simulink model "MaxPilot"  (R2026a)
settings: Solver=VariableStepAuto  StopTime=inf
undefined symbols (not defined in the file or in its folder): f
libraries: instrumentlib x8, slpidlib x4, SignalEditorBlockLib x1
settings Model: Creator=max  LastModifiedBy=Owner

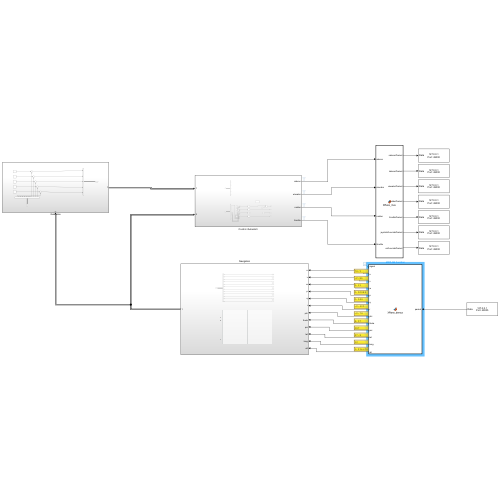
[thumbnail: Simulink's stored preview of the top-level diagram]
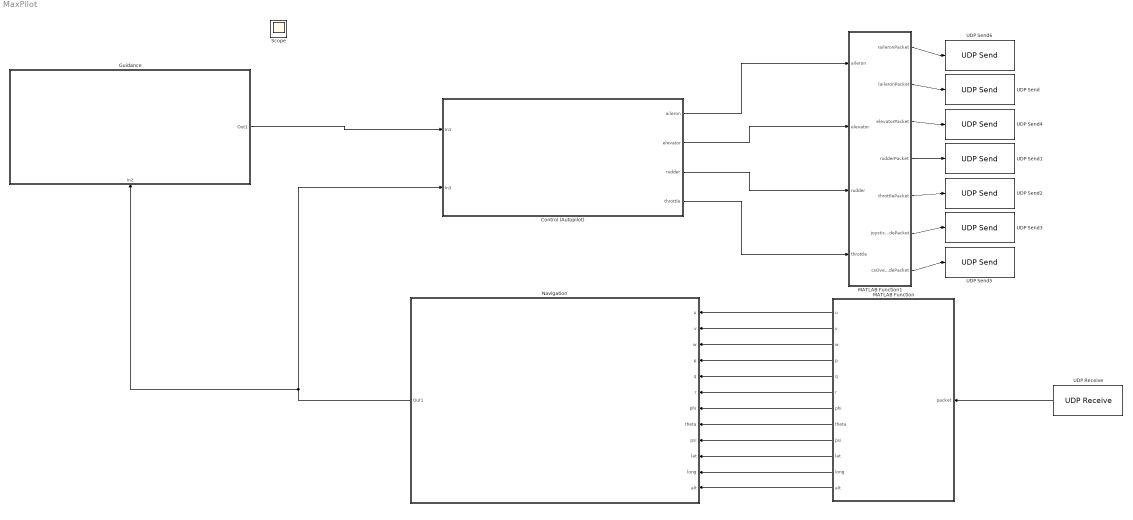
== system MaxPilot ==
  Control (Autopilot) : Subsystem
  Guidance : Subsystem
      settings: PortSchema="{\"entries\":[{\"content\":{\"sides\":[{\"content\":{},\"type\":\"ConnectorPlacement.EquallySpacedRectSide\",\"uuid\":\"e11f845c-727a-4623-8abb-a86b842d9894\"},{\"content\":{\"connectorIds\":[\"Out1\"],\"side\":\"RIGHT\"},\"type\":\"ConnectorPlacement.EquallySpacedRectSide\",\"uuid\":\"0ead8184-70d2-4c1b-98dc-64e560e2a903\"},{\"content\":{\"side\":\"TOP\"},\"type\":\"ConnectorPlacement.EquallySpacedRectSide\",\"uuid\":\"faab937e-1283-4214-83c9-3a230b74f371\"},{\"content\":{\"connectorIds\":[\"In1\"],\"side\":\"BOTTOM\"},\"type\":\"ConnectorPlacement.EquallySpacedRectSide\",\"uuid\":\"89b0e162-5b11-45eb-99f5-a61c863778c0\"}]},\"type\":\"ConnectorPlacement.EquallySpacedConnector\",\"uuid\":\"efd43e26-ed77-40df-bb71-45bc413bd349\"}],\"packageUris\":[\"http://schema.mathworks.com/mf0/Connector/R2020b\"],\"version\":\"1.0\"}"
  MATLAB Function : MATLAB Function  TreatAsAtomicUnit=on
  MATLAB Function1 : MATLAB Function  TreatAsAtomicUnit=on
  Navigation : Subsystem
  UDP Receive : instrumentlib/UDP Receive  LocalAddress=127.0.0.1  LocalPort=49005  EnablePortSharing=off  Host=localhost  Port=9090  GetLatestData=on  DataSize=[ 185, 1 ]  DataType=uint8  ASCIIFormatting=%f,  Terminator=LF  CustomTerminator=10  ByteOrder=big-endian  EnableBlockingMode=on  Timeout=10  SampleTime=0.02  SimulateUsing=Interpreted execution
  UDP Send{,1..6} (7 alike) : instrumentlib/UDP Send  Host=127.0.0.1  Port=49000  LocalAddress=0.0.0.0  LocalPort=-1  EnablePortSharing=off  OutputDatagramPacketSize=509  ByteOrder=big-endian  EnableBlockingMode=on  SimulateUsing=Interpreted execution
  Scope : Scope
      settings: ActiveDisplayYMinimum=-1  ActiveDisplayYMaximum=1
  wires:
  Guidance/1(Out1) -> Control (Autopilot)/1(In1)
  Navigation/1(Out1) -> Control (Autopilot)/2(In3), Guidance/1(In2)
  UDP Receive/1 -> MATLAB Function/1(packet)
  MATLAB Function1/2(laileronPacket) -> UDP Send/1
  MATLAB Function1/3(elevatorPacket) -> UDP Send4/1
  MATLAB Function1/5(throttlePacket) -> UDP Send2/1
  MATLAB Function1/6(joystickOverridePacket) -> UDP Send3/1
  MATLAB Function1/4(rudderPacket) -> UDP Send1/1
  MATLAB Function1/7(csOverridePacket) -> UDP Send5/1
  MATLAB Function1/1(raileronPacket) -> UDP Send6/1
  Control (Autopilot)/1(aileron) -> MATLAB Function1/1(aileron)
  Control (Autopilot)/2(elevator) -> MATLAB Function1/2(elevator)
  Control (Autopilot)/3(rudder) -> MATLAB Function1/3(rudder)
  Control (Autopilot)/4(throttle) -> MATLAB Function1/4(throttle)
  MATLAB Function/2(v) -> Navigation/2(v)
  MATLAB Function/3(w) -> Navigation/3(w)
  MATLAB Function/4(p) -> Navigation/4(p)
  MATLAB Function/5(q) -> Navigation/5(q)
  MATLAB Function/6(r) -> Navigation/6(r)
  MATLAB Function/7(phi) -> Navigation/7(phi)
  MATLAB Function/8(theta) -> Navigation/8(theta)
  MATLAB Function/9(psi) -> Navigation/9(psi)
  MATLAB Function/10(lat) -> Navigation/10(lat)
  MATLAB Function/11(long) -> Navigation/11(long)
  MATLAB Function/12(alt) -> Navigation/12(alt)
  MATLAB Function/1(u) -> Navigation/1(u)

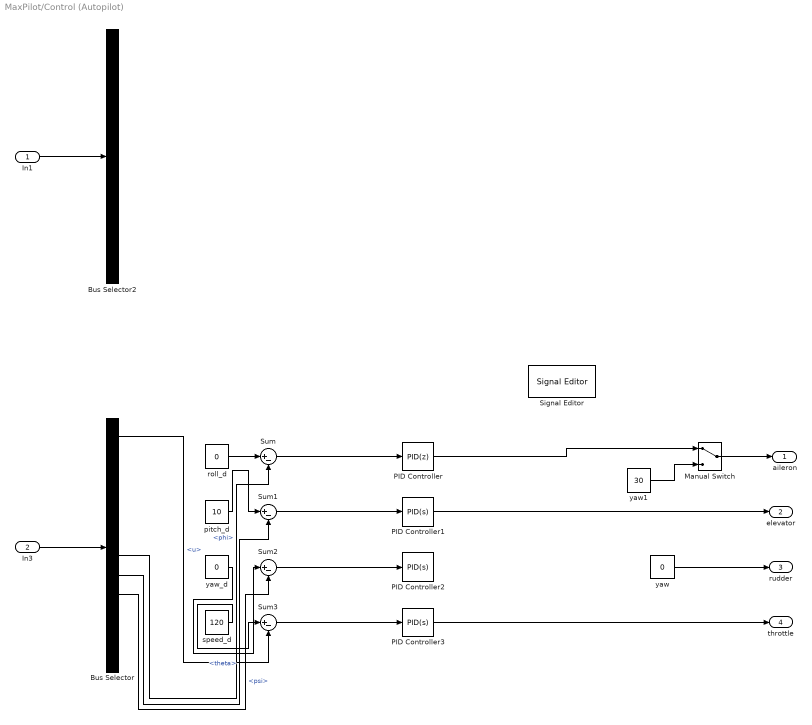
== system MaxPilot/Control (Autopilot) ==
  In1 : Inport
  In3 : Inport  Port=2
  Bus Selector : BusSelector  OutputSignals=u,v,w,p,q,r,phi,theta,psi,lat,long,alt
  Bus Selector2 : BusSelector  OutputSignals=psi_e,North_e,East_e,alt_e,u_e
  Manual Switch : ManualSwitch
  PID Controller : slpidlib/PID Controller  Controller=PID  Form=Parallel  TimeDomain=Discrete-time  UseExternalTs=off  SampleTime=-1  IntegratorMethod=Forward Euler  FilterMethod=Forward Euler  ControllerParametersSource=internal  P=1  I=0  UseKiTs=off  D=0  UseExternalDerivativeSource=off  N=100  UseFilter=on  TunerSelectOption=Frequency Response Based  ZeroCross=off  InitialConditionSource=internal  InitialConditionForIntegrator=0  InitialConditionForFilter=0  DifferentiatorICPrevScaledInput=0  ExternalReset=none  TrackingMode=off  Kt=1  LimitOutput=on  SatLimitsSource=internal  UpperSaturationLimit=10  LowerSaturationLimit=-10  LinearizeAsGain=on  AntiWindupMode=none  Kb=1  LimitIntegrator=off  UpperIntegratorSaturationLimit=inf  LowerIntegratorSaturationLimit=-inf  POutMin=[]  POutMax=[]  IOutMin=[]  IOutMax=[]  DOutMin=[]  DOutMax=[]  NOutMin=[]  NOutMax=[]  SumOutMin=[]  SumOutMax=[]  SaturationOutMin=[]  SaturationOutMax=[]  PParamMin=[]  PParamMax=[]  IParamMin=[]  IParamMax=[]  DParamMin=[]  DParamMax=[]  NParamMin=[]  NParamMax=[]  KbParamMin=[]  KbParamMax=[]  KtParamMin=[]  KtParamMax=[]  KbOutMin=[]  KbOutMax=[]  KtOutMin=[]  KtOutMax=[]  IntegratorOutMin=[]  IntegratorOutMax=[]  FilterOutMin=[]  FilterOutMax=[]  SumI1OutMin=[]  SumI1OutMax=[]  SumI2OutMin=[]  SumI2OutMax=[]  SumI3OutMin=[]  SumI3OutMax=[]  SumI4OutMin=[]  SumI4OutMax=[]  SumDOutMin=[]  SumDOutMax=[]  DifferentiatorOutMin=[]  DifferentiatorOutMax=[]  FilterDiffOutCoefMin=[]  FilterDiffOutCoefMax=[]  ReciprocalOutMin=[]  ReciprocalOutMax=[]  SumDenOutMin=[]  SumDenOutMax=[]  SumNumOutMin=[]  SumNumOutMax=[]  DivideOutMin=[]  DivideOutMax=[]  UdiffTsProdOutMin=[]  UdiffTsProdOutMax=[]  NTsProdOutMin=[]  NTsProdOutMax=[]  UintegralTsProdOutMin=[]  UintegralTsProdOutMax=[]  UngainTsProdOutMin=[]  UngainTsProdOutMax=[]  ClampingZeroOutDataTypeStr=Inherit: Inherit via back propagation  ClampingZeroOutMin=[]  ClampingZeroOutMax=[]  FilterDenConstantOutDataTypeStr=Inherit: Inherit via back propagation  FilterDenConstantOutMin=[]  FilterDenConstantOutMax=[]  PCopyOutDataTypeStr=Inherit: Inherit via back propagation  PCopyOutMin=[]  PCopyOutMax=[]  NCopyOutDataTypeStr=Inherit: Inherit via back propagation  NCopyOutMin=[]  NCopyOutMax=[]  IntegratorContinuousStateAttributes=''  IntegratorStateMustResolveToSignalObject=off  IntegratorRTWStateStorageClass=Auto  FilterContinuousStateAttributes=''  FilterStateMustResolveToSignalObject=off  FilterRTWStateStorageClass=Auto  ParallelPVariant=InternalParameters  IdealPVariant=Disabled  IVariant=InternalParameters  DVariant=InternalParameters  IntegratorVariant=Discrete  SatVariant=Enabled  AWVariant=Passthrough  PCopyVariant=Disabled  TRVariant=Disabled  FdbkBlocksVariant=Forward  IdealPFdbkVariant=Disabled  SatFdbkVariant=Disabled  DerivativeFilterVariant=ForwardEulerFilter  NVariant=InternalParameters  NCopyVariant=Disabled  FilterICVariant=InternalICsFilter  IntegratorICVariant=InternalICs  ExternalResetVariant=Disabled  TRSumVariant=Passthrough  SumFdbkVariant=Disabled  SumVariant=Sum_PID  TsampFilterVariant=InternalTs  TsampNgainVariant=Passthrough  TsampIntegralVariant=Disabled_SignalSpec  ExternalSaturationOutDataTypeStr=Inherit: Same as second input  DerivativeSourceVariant=ErrorSignal  PreIntVariant=InternalPreInt
  PID Controller1 : slpidlib/PID Controller  Controller=PID  Form=Parallel  TimeDomain=Continuous-time  UseExternalTs=off  SampleTime=-1  IntegratorMethod=Forward Euler  FilterMethod=Forward Euler  ControllerParametersSource=internal  P=0.75  I=0  UseKiTs=off  D=0  UseExternalDerivativeSource=off  N=100  UseFilter=on  TunerSelectOption=Transfer Function Based (PID Tuner App)  InitialConditionSource=internal  InitialConditionForIntegrator=0  InitialConditionForFilter=0  DifferentiatorICPrevScaledInput=0  ExternalReset=none  TrackingMode=off  Kt=1  LimitOutput=on  SatLimitsSource=internal  UpperSaturationLimit=20  LowerSaturationLimit=-25  LinearizeAsGain=on  AntiWindupMode=none  Kb=1  LimitIntegrator=off  UpperIntegratorSaturationLimit=inf  LowerIntegratorSaturationLimit=-inf  POutMin=[]  POutMax=[]  IOutMin=[]  IOutMax=[]  DOutMin=[]  DOutMax=[]  NOutMin=[]  NOutMax=[]  SumOutMin=[]  SumOutMax=[]  SaturationOutMin=[]  SaturationOutMax=[]  PParamMin=[]  PParamMax=[]  IParamMin=[]  IParamMax=[]  DParamMin=[]  DParamMax=[]  NParamMin=[]  NParamMax=[]  KbParamMin=[]  KbParamMax=[]  KtParamMin=[]  KtParamMax=[]  KbOutMin=[]  KbOutMax=[]  KtOutMin=[]  KtOutMax=[]  IntegratorOutMin=[]  IntegratorOutMax=[]  FilterOutMin=[]  FilterOutMax=[]  SumI1OutMin=[]  SumI1OutMax=[]  SumI2OutMin=[]  SumI2OutMax=[]  SumI3OutMin=[]  SumI3OutMax=[]  SumI4OutMin=[]  SumI4OutMax=[]  SumDOutMin=[]  SumDOutMax=[]  DifferentiatorOutMin=[]  DifferentiatorOutMax=[]  FilterDiffOutCoefMin=[]  FilterDiffOutCoefMax=[]  ReciprocalOutMin=[]  ReciprocalOutMax=[]  SumDenOutMin=[]  SumDenOutMax=[]  SumNumOutMin=[]  SumNumOutMax=[]  DivideOutMin=[]  DivideOutMax=[]  UdiffTsProdOutMin=[]  UdiffTsProdOutMax=[]  NTsProdOutMin=[]  NTsProdOutMax=[]  UintegralTsProdOutMin=[]  UintegralTsProdOutMax=[]  UngainTsProdOutMin=[]  UngainTsProdOutMax=[]  ClampingZeroOutDataTypeStr=Inherit: Inherit via back propagation  ClampingZeroOutMin=[]  ClampingZeroOutMax=[]  FilterDenConstantOutDataTypeStr=Inherit: Inherit via back propagation  FilterDenConstantOutMin=[]  FilterDenConstantOutMax=[]  PCopyOutDataTypeStr=Inherit: Inherit via back propagation  PCopyOutMin=[]  PCopyOutMax=[]  NCopyOutDataTypeStr=Inherit: Inherit via back propagation  NCopyOutMin=[]  NCopyOutMax=[]  IntegratorContinuousStateAttributes=''  IntegratorStateMustResolveToSignalObject=off  IntegratorRTWStateStorageClass=Auto  FilterContinuousStateAttributes=''  FilterStateMustResolveToSignalObject=off  FilterRTWStateStorageClass=Auto  ParallelPVariant=InternalParameters  IdealPVariant=Disabled  IVariant=InternalParameters  DVariant=InternalParameters  IntegratorVariant=Continuous  SatVariant=Enabled  AWVariant=Passthrough  PCopyVariant=Disabled  TRVariant=Disabled  FdbkBlocksVariant=Forward  IdealPFdbkVariant=Disabled  SatFdbkVariant=Disabled  DerivativeFilterVariant=ContFilter  NVariant=InternalParameters  NCopyVariant=Disabled  FilterICVariant=InternalICsFilter  IntegratorICVariant=InternalICs  ExternalResetVariant=Disabled  TRSumVariant=Passthrough  SumFdbkVariant=Disabled  SumVariant=Sum_PID  TsampFilterVariant=InternalTs  TsampNgainVariant=Passthrough  TsampIntegralVariant=Disabled_SignalSpec  ExternalSaturationOutDataTypeStr=Inherit: Same as second input  DerivativeSourceVariant=ErrorSignal  PreIntVariant=InternalPreInt
  PID Controller2 : slpidlib/PID Controller  Controller=PID  Form=Parallel  TimeDomain=Continuous-time  UseExternalTs=off  SampleTime=-1  IntegratorMethod=Forward Euler  FilterMethod=Forward Euler  ControllerParametersSource=internal  P=1  I=0  UseKiTs=off  D=0  UseExternalDerivativeSource=off  N=100  UseFilter=on  TunerSelectOption=Transfer Function Based (PID Tuner App)  InitialConditionSource=internal  InitialConditionForIntegrator=0  InitialConditionForFilter=0  DifferentiatorICPrevScaledInput=0  ExternalReset=none  TrackingMode=off  Kt=1  LimitOutput=on  SatLimitsSource=internal  UpperSaturationLimit=15  LowerSaturationLimit=-15  LinearizeAsGain=on  AntiWindupMode=none  Kb=1  LimitIntegrator=off  UpperIntegratorSaturationLimit=inf  LowerIntegratorSaturationLimit=-inf  POutMin=[]  POutMax=[]  IOutMin=[]  IOutMax=[]  DOutMin=[]  DOutMax=[]  NOutMin=[]  NOutMax=[]  SumOutMin=[]  SumOutMax=[]  SaturationOutMin=[]  SaturationOutMax=[]  PParamMin=[]  PParamMax=[]  IParamMin=[]  IParamMax=[]  DParamMin=[]  DParamMax=[]  NParamMin=[]  NParamMax=[]  KbParamMin=[]  KbParamMax=[]  KtParamMin=[]  KtParamMax=[]  KbOutMin=[]  KbOutMax=[]  KtOutMin=[]  KtOutMax=[]  IntegratorOutMin=[]  IntegratorOutMax=[]  FilterOutMin=[]  FilterOutMax=[]  SumI1OutMin=[]  SumI1OutMax=[]  SumI2OutMin=[]  SumI2OutMax=[]  SumI3OutMin=[]  SumI3OutMax=[]  SumI4OutMin=[]  SumI4OutMax=[]  SumDOutMin=[]  SumDOutMax=[]  DifferentiatorOutMin=[]  DifferentiatorOutMax=[]  FilterDiffOutCoefMin=[]  FilterDiffOutCoefMax=[]  ReciprocalOutMin=[]  ReciprocalOutMax=[]  SumDenOutMin=[]  SumDenOutMax=[]  SumNumOutMin=[]  SumNumOutMax=[]  DivideOutMin=[]  DivideOutMax=[]  UdiffTsProdOutMin=[]  UdiffTsProdOutMax=[]  NTsProdOutMin=[]  NTsProdOutMax=[]  UintegralTsProdOutMin=[]  UintegralTsProdOutMax=[]  UngainTsProdOutMin=[]  UngainTsProdOutMax=[]  ClampingZeroOutDataTypeStr=Inherit: Inherit via back propagation  ClampingZeroOutMin=[]  ClampingZeroOutMax=[]  FilterDenConstantOutDataTypeStr=Inherit: Inherit via back propagation  FilterDenConstantOutMin=[]  FilterDenConstantOutMax=[]  PCopyOutDataTypeStr=Inherit: Inherit via back propagation  PCopyOutMin=[]  PCopyOutMax=[]  NCopyOutDataTypeStr=Inherit: Inherit via back propagation  NCopyOutMin=[]  NCopyOutMax=[]  IntegratorContinuousStateAttributes=''  IntegratorStateMustResolveToSignalObject=off  IntegratorRTWStateStorageClass=Auto  FilterContinuousStateAttributes=''  FilterStateMustResolveToSignalObject=off  FilterRTWStateStorageClass=Auto  ParallelPVariant=InternalParameters  IdealPVariant=Disabled  IVariant=InternalParameters  DVariant=InternalParameters  IntegratorVariant=Continuous  SatVariant=Enabled  AWVariant=Passthrough  PCopyVariant=Disabled  TRVariant=Disabled  FdbkBlocksVariant=Forward  IdealPFdbkVariant=Disabled  SatFdbkVariant=Disabled  DerivativeFilterVariant=ContFilter  NVariant=InternalParameters  NCopyVariant=Disabled  FilterICVariant=InternalICsFilter  IntegratorICVariant=InternalICs  ExternalResetVariant=Disabled  TRSumVariant=Passthrough  SumFdbkVariant=Disabled  SumVariant=Sum_PID  TsampFilterVariant=InternalTs  TsampNgainVariant=Passthrough  TsampIntegralVariant=Disabled_SignalSpec  ExternalSaturationOutDataTypeStr=Inherit: Same as second input  DerivativeSourceVariant=ErrorSignal  PreIntVariant=InternalPreInt
  PID Controller3 : slpidlib/PID Controller  Controller=PID  Form=Parallel  TimeDomain=Continuous-time  UseExternalTs=off  SampleTime=-1  IntegratorMethod=Forward Euler  FilterMethod=Forward Euler  ControllerParametersSource=internal  P=0.1  I=0  UseKiTs=off  D=0  UseExternalDerivativeSource=off  N=100  UseFilter=on  TunerSelectOption=Transfer Function Based (PID Tuner App)  InitialConditionSource=internal  InitialConditionForIntegrator=0  InitialConditionForFilter=0  DifferentiatorICPrevScaledInput=0  ExternalReset=none  TrackingMode=off  Kt=1  LimitOutput=on  SatLimitsSource=internal  UpperSaturationLimit=1  LowerSaturationLimit=0  LinearizeAsGain=on  AntiWindupMode=none  Kb=1  LimitIntegrator=off  UpperIntegratorSaturationLimit=inf  LowerIntegratorSaturationLimit=-inf  POutMin=[]  POutMax=[]  IOutMin=[]  IOutMax=[]  DOutMin=[]  DOutMax=[]  NOutMin=[]  NOutMax=[]  SumOutMin=[]  SumOutMax=[]  SaturationOutMin=[]  SaturationOutMax=[]  PParamMin=[]  PParamMax=[]  IParamMin=[]  IParamMax=[]  DParamMin=[]  DParamMax=[]  NParamMin=[]  NParamMax=[]  KbParamMin=[]  KbParamMax=[]  KtParamMin=[]  KtParamMax=[]  KbOutMin=[]  KbOutMax=[]  KtOutMin=[]  KtOutMax=[]  IntegratorOutMin=[]  IntegratorOutMax=[]  FilterOutMin=[]  FilterOutMax=[]  SumI1OutMin=[]  SumI1OutMax=[]  SumI2OutMin=[]  SumI2OutMax=[]  SumI3OutMin=[]  SumI3OutMax=[]  SumI4OutMin=[]  SumI4OutMax=[]  SumDOutMin=[]  SumDOutMax=[]  DifferentiatorOutMin=[]  DifferentiatorOutMax=[]  FilterDiffOutCoefMin=[]  FilterDiffOutCoefMax=[]  ReciprocalOutMin=[]  ReciprocalOutMax=[]  SumDenOutMin=[]  SumDenOutMax=[]  SumNumOutMin=[]  SumNumOutMax=[]  DivideOutMin=[]  DivideOutMax=[]  UdiffTsProdOutMin=[]  UdiffTsProdOutMax=[]  NTsProdOutMin=[]  NTsProdOutMax=[]  UintegralTsProdOutMin=[]  UintegralTsProdOutMax=[]  UngainTsProdOutMin=[]  UngainTsProdOutMax=[]  ClampingZeroOutDataTypeStr=Inherit: Inherit via back propagation  ClampingZeroOutMin=[]  ClampingZeroOutMax=[]  FilterDenConstantOutDataTypeStr=Inherit: Inherit via back propagation  FilterDenConstantOutMin=[]  FilterDenConstantOutMax=[]  PCopyOutDataTypeStr=Inherit: Inherit via back propagation  PCopyOutMin=[]  PCopyOutMax=[]  NCopyOutDataTypeStr=Inherit: Inherit via back propagation  NCopyOutMin=[]  NCopyOutMax=[]  IntegratorContinuousStateAttributes=''  IntegratorStateMustResolveToSignalObject=off  IntegratorRTWStateStorageClass=Auto  FilterContinuousStateAttributes=''  FilterStateMustResolveToSignalObject=off  FilterRTWStateStorageClass=Auto  ParallelPVariant=InternalParameters  IdealPVariant=Disabled  IVariant=InternalParameters  DVariant=InternalParameters  IntegratorVariant=Continuous  SatVariant=Enabled  AWVariant=Passthrough  PCopyVariant=Disabled  TRVariant=Disabled  FdbkBlocksVariant=Forward  IdealPFdbkVariant=Disabled  SatFdbkVariant=Disabled  DerivativeFilterVariant=ContFilter  NVariant=InternalParameters  NCopyVariant=Disabled  FilterICVariant=InternalICsFilter  IntegratorICVariant=InternalICs  ExternalResetVariant=Disabled  TRSumVariant=Passthrough  SumFdbkVariant=Disabled  SumVariant=Sum_PID  TsampFilterVariant=InternalTs  TsampNgainVariant=Passthrough  TsampIntegralVariant=Disabled_SignalSpec  ExternalSaturationOutDataTypeStr=Inherit: Same as second input  DerivativeSourceVariant=ErrorSignal  PreIntVariant=InternalPreInt
  Signal Editor : SignalEditorBlockLib/Signal Editor  FileName=C:\Users\Owner\ws\MaxPilot\sw\systemIdSignals.mat  ActiveScenario=systemID  ActiveSignal=doublet  IsBus=off  OutputBusObjectStr=Bus: BusObject  SampleTime=0  ZeroCross=off  OutputAfterFinalValue=Setting to zero  Unit=inherit  PreserveSignalName=on  ApplySigPropsToAllScenarios=on  ApplySigPropsToAllSignals=off  SignalPropertySource=Dialog parameters
  Sum{,1..3} (4 alike) : Sum  Inputs=|+-
  pitch_d : Constant  Value=10
  roll_d : Constant  Value=0
  speed_d : Constant  Value=120
  yaw : Constant  Value=0
  yaw1 : Constant  Value=30
  yaw_d : Constant  Value=0
  aileron : Outport
  elevator : Outport  Port=2
  rudder : Outport  Port=3
  throttle : Outport  Port=4
  wires:
  In3/1 -> Bus Selector/1
  In1/1 -> Bus Selector2/1
  Sum1/1 -> PID Controller1/1
  Sum2/1 -> PID Controller2/1
  Sum3/1 -> PID Controller3/1
  PID Controller3/1 -> throttle/1
  Bus Selector/8 -> Sum1/2  "<theta>"
  pitch_d/1 -> Sum1/1
  Bus Selector/7 -> Sum/2  "<phi>"
  roll_d/1 -> Sum/1
  Bus Selector/9 -> Sum2/2  "<psi>"
  yaw_d/1 -> Sum2/1
  speed_d/1 -> Sum3/1
  Bus Selector/1 -> Sum3/2  "<u>"
  Sum/1 -> PID Controller/1
  PID Controller1/1 -> elevator/1
  PID Controller/1 -> Manual Switch/1
  Manual Switch/1 -> aileron/1
  yaw1/1 -> Manual Switch/2
  yaw/1 -> rudder/1

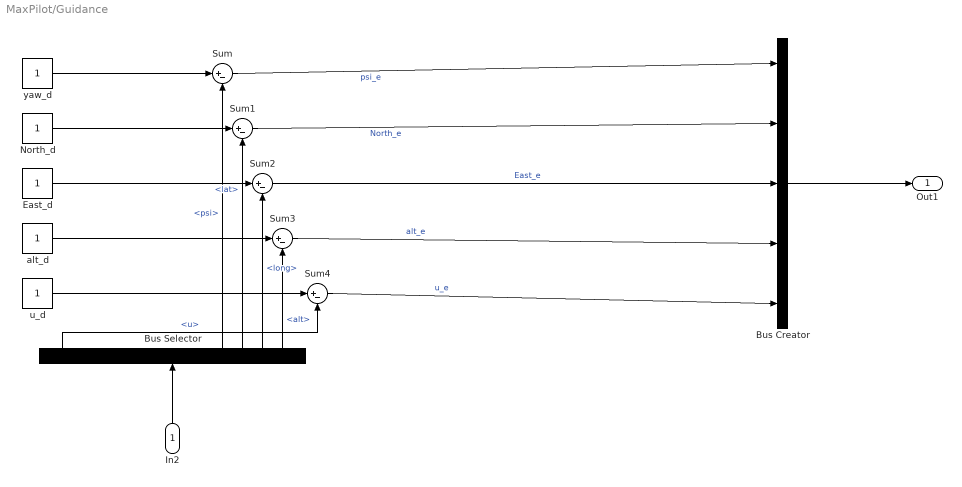
== system MaxPilot/Guidance ==
  In2 : Inport
  Bus Creator : BusCreator  Inputs=5
  Bus Selector : BusSelector  OutputSignals=u,v,w,p,q,r,phi,theta,psi,lat,long,alt
  East_d : Constant
  North_d : Constant
  Sum{,1..4} (5 alike) : Sum  Inputs=|+-
  alt_d : Constant
  u_d : Constant
  yaw_d : Constant
  Out1 : Outport
  wires:
  In2/1 -> Bus Selector/1
  Bus Creator/1 -> Out1/1
  Bus Selector/12 -> Sum3/2  "<alt>"
  Bus Selector/11 -> Sum2/2  "<long>"
  Bus Selector/10 -> Sum1/2  "<lat>"
  Bus Selector/9 -> Sum/2  "<psi>"
  alt_d/1 -> Sum3/1
  East_d/1 -> Sum2/1
  North_d/1 -> Sum1/1
  yaw_d/1 -> Sum/1
  Sum/1 -> Bus Creator/1  "psi_e"
  Sum1/1 -> Bus Creator/2  "North_e"
  Sum2/1 -> Bus Creator/3  "East_e"
  Sum3/1 -> Bus Creator/4  "alt_e"
  Bus Selector/1 -> Sum4/2  "<u>"
  u_d/1 -> Sum4/1
  Sum4/1 -> Bus Creator/5  "u_e"

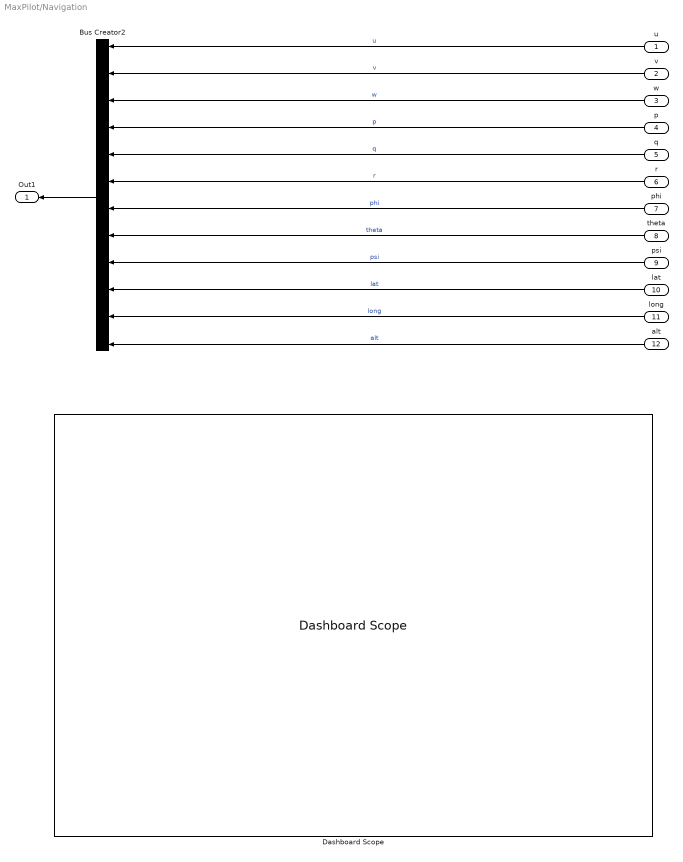
== system MaxPilot/Navigation ==
  u : Inport
  v : Inport  Port=2
  w : Inport  Port=3
  p : Inport  Port=4
  q : Inport  Port=5
  r : Inport  Port=6
  phi : Inport  Port=7
  theta : Inport  Port=8
  psi : Inport  Port=9
  lat : Inport  Port=10
  long : Inport  Port=11
  alt : Inport  Port=12
  Bus Creator2 : BusCreator  Inputs=12
  Dashboard Scope : DashboardScope  FontColor=[0.0, 0.0, 0.0]
  Out1 : Outport
  wires:
  Bus Creator2/1 -> Out1/1
  u/1 -> Bus Creator2/1  "u"
  v/1 -> Bus Creator2/2  "v"
  w/1 -> Bus Creator2/3  "w"
  p/1 -> Bus Creator2/4  "p"
  q/1 -> Bus Creator2/5  "q"
  r/1 -> Bus Creator2/6  "r"
  phi/1 -> Bus Creator2/7  "phi"
  theta/1 -> Bus Creator2/8  "theta"
  psi/1 -> Bus Creator2/9  "psi"
  lat/1 -> Bus Creator2/10  "lat"
  long/1 -> Bus Creator2/11  "long"
  alt/1 -> Bus Creator2/12  "alt"

== matlab function MaxPilot/MATLAB Function1 ==
  data: raileronPacket output; aileron input; laileronPacket output; elevator input; rudder input; throttle input; elevatorPacket output; rudderPacket output; throttlePacket output; joystickOverridePacket output; csOverridePacket output
function  [raileronPacket, laileronPacket, elevatorPacket, rudderPacket, throttlePacket, joystickOverridePacket, csOverridePacket] = XPlane_mux(aileron, elevator, rudder, throttle)

% X-Plane DREF packet builder
%
% Input:
% u(1) = aileron     (-10 to 10)
% u(2) = elevator    (-25 to 20)
% u(3) = rudder      (-15 to 15)
% u(4) = throttle    (0 to 1)
%
% Output:
% packet = UDP byte stream

% Datarefs
drefs = {
    'sim/operation/override/override_joystick'
    'sim/operation/override/override_control_surfaces'
    'sim/flightmodel2/wing/aileron1_deg[2]'
    'sim/flightmodel2/wing/aileron1_deg[3]'
    'sim/flightmodel2/wing/elevator1_deg[8]'
    'sim/flightmodel2/wing/rudder1_deg[10]'
    'sim/cockpit2/engine/actuators/throttle_ratio_all'
    };

% Values
values = [
    single(1)
    single(1)
    single(aileron)
    single(-aileron)
    single(-elevator)
    single(rudder)
    single(throttle)
    ];

indices = [
    0;  % override joystick
    8;  % override surfaces
    0;  % raileron
    1;  % laileron
    8;  % elevator
    10;  % rudder
    0;  % throttle
];

for k = 1:length(drefs)
    packet = zeros(509,1,'uint8');
    packet(1:5) = uint8('DREF0');
    packet(6:9) = typecast(values(k),'uint8');
    name = uint8(drefs{k});
    packet(10:9+length(name)) = name;

    switch k
        case 1
            joystickOverridePacket = packet;
        case 2
            csOverridePacket = packet;
        case 3
            raileronPacket = packet;
        case 4
            laileronPacket = packet;
        case 5
            elevatorPacket = packet;
        case 6
            rudderPacket = packet;
        case 7
            throttlePacket = packet;
    end
end

== matlab function MaxPilot/MATLAB Function ==
  data: packet input; u output; v output; w output; p output; q output; r output; phi output; theta output; psi output; lat output; long output; alt output
 function [u, v, w, ...
        p, q, r,...
        phi, theta, psi, ...
        lat, long, alt]...
          = XPlane_demux(packet)

% init
u = single(0);
v = single(0);
w = single(0);
p = single(0);
q = single(0);
r = single(0);
phi = single(0);
theta = single(0);
psi = single(0);
lat = single(0);
long = single(0);
alt = single(0);

% Speeds
airspeed = single(0);

% Pitch, roll, & headings
pitch = single(0);
roll = single(0);
hding_true = single(0);
% hding_mag = single(0);

% Angular velocities
% roll_torque = single(0);
% pitch_torque = single(0);
% yaw_torque = single(0);
pitch_rate = single(0);
roll_rate = single(0);
yaw_rate = single(0);

% Angle of attack, sideslip, and paths
alpha = single(0);
beta = single(0);
% hpath = single(0);
% vpath = single(0);
% slip = single(0);

if ~(packet(1)=='D' && packet(2)=='A' && packet(3)=='T' && packet(4)=='A')
    return;
end

payload = packet(6:end);
N = floor(length(payload)/36);

for k = 1:N
    offset = (k-1)*36;
    idx = typecast(uint8(payload(offset+1:offset+4)),'int32');
    values = typecast(uint8(payload(offset+5:offset+36)),'single');

    switch idx
        % Speeds
        case 3
            airspeed = values(1);

        % Angular velocities
        case 16
            pitch_rate = values(1);
            roll_rate = values(2);
            yaw_rate = values(3);

        % Pitch, roll & heading
        case 17
            pitch = values(1);
            roll = values(2);
            hding_true = values(3);
            % hding_mag = values(4);

        % Angle of attack, sideslip, and paths
        case 18
            alpha = values(1);
            beta = values(2);
            % hpath = values(3);
            % vpath = values(4);
            % slip = values(5);

       % Latitude, longitude, & altitude
        case 20
            lat = values(1);
            long = values(2);
            alt = values(3);
    end
end

u = airspeed * cos(pi/180 * alpha) * cos(pi/180 * beta);
v = airspeed * sin(pi/180 * beta);
w = airspeed * sin(pi/180 * alpha) * cos(pi/180 * beta);
p = roll_rate;
q = pitch_rate;
r = yaw_rate;
phi = roll;
theta = pitch;
psi = hding_true;
